simulink model "watertankPI_cmp"  (R2026a)
settings: Solver=ode45  StopTime=Tf  EnableMultiTasking=on
values from neighbouring files (symbols this model uses):
  Ts = 1    [DA2_main.m]    (also in LSTMController.m; TunePIControllerWithReinforcementLearningExample.m; build_compare_model.m)
undefined symbols (not defined in the file or in its folder): DiscIntNeverNeededParam
libraries: simulink x1, slpidlib x1
settings Model: Creator=The MathWorks, Inc.  LastModifiedBy=Dharu
settings DataIOCC: SignalLoggingName=logsOut
settings OptimizationCC: InitFltsAndDblsToZero=on
settings DebuggingCC: SaveWithParameterizedLinksMsg=none  SignalResolutionControl=TryResolveAllWithWarning  MultiTaskDSMMsg=warning
settings HardwareCC: ProdHWDeviceType=Specified
settings GRTTargetCC: TargetFcnLib=ansi_tfl_tmw.mat  CombineOutputUpdateFcns=off  GRTInterface=on

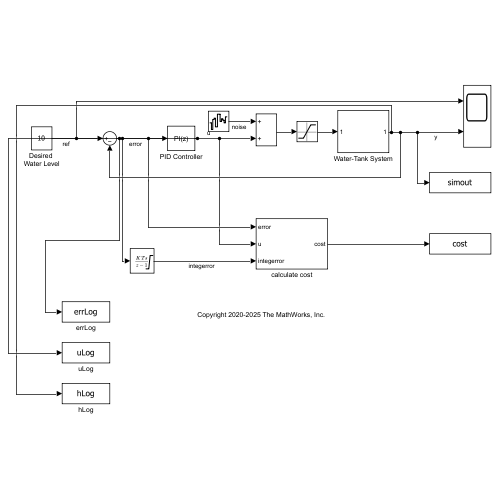
[thumbnail: Simulink's stored preview of the top-level diagram]
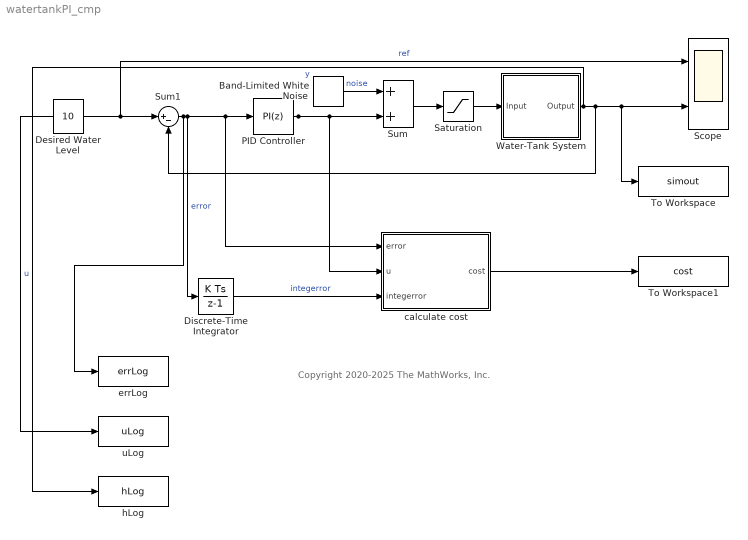
== system watertankPI_cmp ==
  note: Copyright 2020-2025 The MathWorks, Inc.
  Band-Limited White Noise : simulink/Sources/Band-Limited White Noise  Cov=0.01  Ts=Ts  seed=[23341]
  Desired Water Level : Constant  Value=10
  Discrete-Time Integrator : DiscreteIntegrator  gainval=1  SampleTime=Ts  LimitOutput=on  UpperSaturationLimit=100  LowerSaturationLimit=-100  ICPrevOutput=DiscIntNeverNeededParam  ICPrevScaledInput=DiscIntNeverNeededParam
  PID Controller : slpidlib/PID Controller  Tag=PID1  Controller=PI  Form=Parallel  TimeDomain=Discrete-time  UseExternalTs=off  SampleTime=Ts  IntegratorMethod=Forward Euler  FilterMethod=Forward Euler  ControllerParametersSource=internal  P=3.4373  I=0.035778  UseKiTs=off  D=-7.525674  UseExternalDerivativeSource=off  N=0.201208  UseFilter=on  TunerSelectOption=Transfer Function Based (PID Tuner App)  ZeroCross=off  InitialConditionSource=internal  InitialConditionForIntegrator=0  InitialConditionForFilter=0  DifferentiatorICPrevScaledInput=0  ExternalReset=none  TrackingMode=off  Kt=1  LimitOutput=off  SatLimitsSource=internal  UpperSaturationLimit=inf  LowerSaturationLimit=-inf  LinearizeAsGain=off  AntiWindupMode=none  Kb=1  LimitIntegrator=off  UpperIntegratorSaturationLimit=inf  LowerIntegratorSaturationLimit=-inf  POutMin=[ ]  POutMax=[ ]  IOutMin=[ ]  IOutMax=[ ]  DOutMin=[ ]  DOutMax=[ ]  NOutMin=[ ]  NOutMax=[ ]  SumOutMin=[ ]  SumOutMax=[ ]  SaturationOutMin=[ ]  SaturationOutMax=[ ]  PParamMin=[ ]  PParamMax=[ ]  IParamMin=[ ]  IParamMax=[ ]  DParamMin=[ ]  DParamMax=[ ]  NParamMin=[ ]  NParamMax=[ ]  KbParamMin=[ ]  KbParamMax=[ ]  KtParamMin=[ ]  KtParamMax=[ ]  KbOutMin=[ ]  KbOutMax=[ ]  KtOutMin=[ ]  KtOutMax=[ ]  IntegratorOutMin=[ ]  IntegratorOutMax=[ ]  FilterOutMin=[ ]  FilterOutMax=[ ]  SumI1OutMin=[ ]  SumI1OutMax=[ ]  SumI2OutMin=[ ]  SumI2OutMax=[ ]  SumI3OutMin=[ ]  SumI3OutMax=[ ]  SumI4OutMin=[]  SumI4OutMax=[]  SumDOutMin=[ ]  SumDOutMax=[ ]  DifferentiatorOutMin=[]  DifferentiatorOutMax=[]  FilterDiffOutCoefMin=[]  FilterDiffOutCoefMax=[]  ReciprocalOutMin=[]  ReciprocalOutMax=[]  SumDenOutMin=[]  SumDenOutMax=[]  SumNumOutMin=[]  SumNumOutMax=[]  DivideOutMin=[]  DivideOutMax=[]  UdiffTsProdOutMin=[]  UdiffTsProdOutMax=[]  NTsProdOutMin=[]  NTsProdOutMax=[]  UintegralTsProdOutMin=[]  UintegralTsProdOutMax=[]  UngainTsProdOutMin=[]  UngainTsProdOutMax=[]  ClampingZeroOutDataTypeStr=Inherit: Inherit via back propagation  ClampingZeroOutMin=[]  ClampingZeroOutMax=[]  FilterDenConstantOutDataTypeStr=Inherit: Inherit via back propagation  FilterDenConstantOutMin=[]  FilterDenConstantOutMax=[]  PCopyOutDataTypeStr=Inherit: Inherit via back propagation  PCopyOutMin=[]  PCopyOutMax=[]  NCopyOutDataTypeStr=Inherit: Inherit via back propagation  NCopyOutMin=[]  NCopyOutMax=[]  IntegratorContinuousStateAttributes=''  IntegratorStateMustResolveToSignalObject=off  IntegratorRTWStateStorageClass=Auto  FilterContinuousStateAttributes=''  FilterStateMustResolveToSignalObject=off  FilterRTWStateStorageClass=Auto  ParallelPVariant=InternalParameters  IdealPVariant=Disabled  IVariant=InternalParameters  DVariant=Disabled  IntegratorVariant=Discrete  SatVariant=Disabled  AWVariant=Passthrough  PCopyVariant=Disabled  TRVariant=Disabled  FdbkBlocksVariant=Forward  IdealPFdbkVariant=Disabled  SatFdbkVariant=Disabled  DerivativeFilterVariant=Disabled  NVariant=Disabled  NCopyVariant=Disabled_SignalSpec  FilterICVariant=Disabled  IntegratorICVariant=InternalICs  ExternalResetVariant=Disabled  TRSumVariant=Passthrough  SumFdbkVariant=Disabled  SumVariant=Sum_PI  TsampFilterVariant=InternalTs  TsampNgainVariant=Passthrough  TsampIntegralVariant=Disabled_SignalSpec  ExternalSaturationOutDataTypeStr=Inherit: Same as second input  DerivativeSourceVariant=Disabled  PreIntVariant=InternalPreInt
  Saturation : Saturate  UpperLimit=12  LowerLimit=0
  Scope : Scope  NumInputPorts=2
      settings: ActiveDisplayYMinimum=-8.8693854504523131  ActiveDisplayYMaximum=18.205080928572428
  Sum : Sum
  Sum1 : Sum  Inputs=|+-  SaturateOnIntegerOverflow=on
  To Workspace : ToWorkspace  VariableName=simout  SaveFormat=Timeseries  SampleTime=-1
  To Workspace1 : ToWorkspace  VariableName=cost  SaveFormat=Timeseries  SampleTime=-1
  Water-Tank System : Subsystem
  calculate cost : Subsystem
  errLog : ToWorkspace  VariableName=errLog  SaveFormat=Timeseries  SampleTime=Ts
  hLog : ToWorkspace  VariableName=hLog  SaveFormat=Timeseries  SampleTime=Ts
  uLog : ToWorkspace  VariableName=uLog  SaveFormat=Timeseries  SampleTime=Ts
  wires:
  Desired Water Level/1 -> Scope/1, Sum1/1  "ref"
  Sum1/1 -> Discrete-Time Integrator/1, calculate cost/1(error), PID Controller/1, errLog/1  "error"
  Water-Tank System/1(Output) -> To Workspace/1, Scope/2, Sum1/2, hLog/1  "y"
  Sum/1 -> Saturation/1
  PID Controller/1 -> calculate cost/2(u), Sum/2, uLog/1  "u"
  Band-Limited White Noise/1 -> Sum/1  "noise"
  calculate cost/1(cost) -> To Workspace1/1
  Saturation/1 -> Water-Tank System/1(Input)
  Discrete-Time Integrator/1 -> calculate cost/3(integerror)  "integerror"

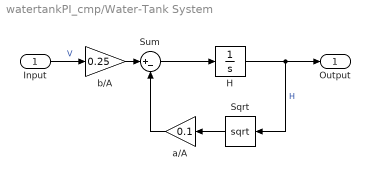
== system watertankPI_cmp/Water-Tank System ==
  Input : Inport
  H : Integrator  InitialCondition=1  LimitOutput=on  LowerSaturationLimit=0
  Sqrt : Sqrt  OutputSignalType=real
  Sum : Sum  Inputs=|+-  SaturateOnIntegerOverflow=on
  a/A : Gain  Gain=0.1  SaturateOnIntegerOverflow=on  OutDataTypeStr=Inherit: Same as input  ParamDataTypeStr=Inherit: Same as input
  b/A : Gain  Gain=0.25  SaturateOnIntegerOverflow=on  OutDataTypeStr=Inherit: Same as input  ParamDataTypeStr=Inherit: Same as input
  Output : Outport  VectorParamsAs1DForOutWhenUnconnected=off
  wires:
  b/A/1 -> Sum/1
  Sum/1 -> H/1
  H/1 -> Sqrt/1, Output/1  "H"
  Sqrt/1 -> a/A/1
  a/A/1 -> Sum/2
  Input/1 -> b/A/1  "V"

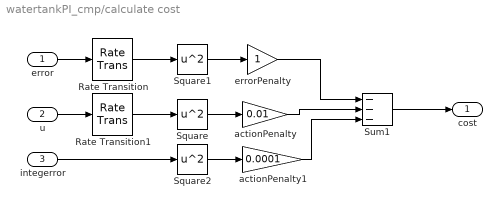
== system watertankPI_cmp/calculate cost ==
  error : Inport
  u : Inport  Port=2
  integerror : Inport  Port=3
  Rate Transition : RateTransition  OutPortSampleTime=Ts
  Rate Transition1 : RateTransition  OutPortSampleTime=Ts
  Square : Math  Operator=square
  Square1 : Math  Operator=square
  Square2 : Math  Operator=square
  Sum1 : Sum  Inputs=---  OutDataTypeStr=double
  actionPenalty : Gain  Gain=0.01
  actionPenalty1 : Gain  Gain=0.0001
  errorPenalty : Gain
  cost : Outport  VectorParamsAs1DForOutWhenUnconnected=off
  wires:
  Square1/1 -> errorPenalty/1
  errorPenalty/1 -> Sum1/1
  actionPenalty/1 -> Sum1/2
  Square/1 -> actionPenalty/1
  u/1 -> Rate Transition1/1
  error/1 -> Rate Transition/1
  Sum1/1 -> cost/1
  Rate Transition/1 -> Square1/1
  Rate Transition1/1 -> Square/1
  integerror/1 -> Square2/1
  actionPenalty1/1 -> Sum1/3
  Square2/1 -> actionPenalty1/1
